simulink model "prob2"  (R2020b)
settings: Solver=VariableStepAuto  StartTime=0.0  StopTime=10.0  RelTol=1e-3
values from neighbouring files (symbols this model uses):
  b = 7500    [values.mat]
  k1 = 35000    [values.mat]
  k2 = 60000    [values.mat]
  M1 = 500    [values.mat]
  M2 = 15    [values.mat]
settings Model: Creator=DELL  LastModifiedBy=DELL

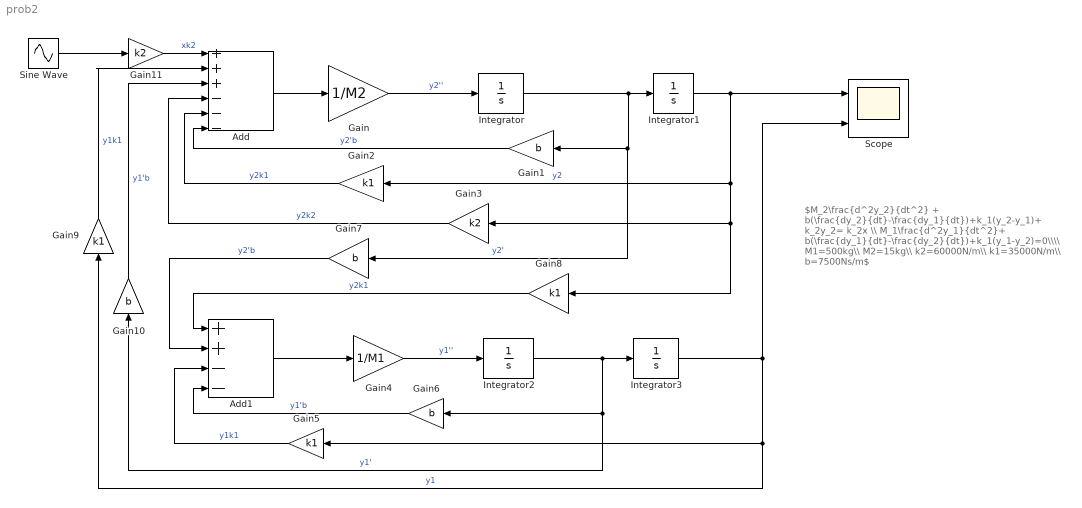
== system prob2 ==
  note: $M_2\frac{d^2y_2}{dt^2} + b(\frac{dy_2}{dt}-\frac{dy_1}{dt})+k_1(y_2-y_1)+ k_2y_2= k_2x \\ M_1\frac{d^2y_1}{dt^2}+ b(\frac{dy_1}{dt}-\frac{dy_2}{dt})+k_1(y_1-y_2)=0\\\\ M1=500kg\\ M2=15kg\\ k2=60000N/m\\ k1=35000N/m\\ b=7500Ns/m$
  Add : Sum  Inputs=+++---
  Add1 : Sum  Inputs=++--
  Gain : Gain  Gain=1/M2
  Gain{1,6..7,10} (4 alike) : Gain  Gain=b
  Gain11 : Gain  Gain=k2
  Gain{2,5,8..9} (4 alike) : Gain  Gain=k1
  Gain3 : Gain  Gain=k2
  Gain4 : Gain  Gain=1/M1
  Integrator{,1..3} (4 alike) : Integrator
  Scope : Scope  NumInputPorts=2
  Sine Wave : Sin  SampleTime=0
  wires:
  Integrator/1 -> Gain7/1, Gain1/1, Integrator1/1  "y2'"
  Gain/1 -> Integrator/1  "y2''"
  Add/1 -> Gain/1
  Integrator1/1 -> Gain8/1, Gain3/1, Gain2/1, Scope/1  "y2"
  Integrator2/1 -> Gain10/1, Gain6/1, Integrator3/1  "y1'"
  Gain4/1 -> Integrator2/1  "y1''"
  Integrator3/1 -> Gain5/1, Gain9/1, Scope/2  "y1"
  Add1/1 -> Gain4/1
  Gain1/1 -> Add/6  "y2'b"
  Gain2/1 -> Add/5  "y2k1"
  Gain3/1 -> Add/4  "y2k2"
  Gain6/1 -> Add1/4  "y1'b"
  Gain5/1 -> Add1/3  "y1k1"
  Sine Wave/1 -> Gain11/1
  Gain7/1 -> Add1/2  "y2'b"
  Gain8/1 -> Add1/1  "y2k1"
  Gain10/1 -> Add/3  "y1'b"
  Gain9/1 -> Add/2  "y1k1"
  Gain11/1 -> Add/1  "xk2"
